simulink model "IIR"  (R2025a)
settings: Solver=ode45  StartTime=0.0  StopTime=10000  RelTol=1e-3  EnableMultiTasking=on
PreLoadFcn:
  | IIR_PreLoadFcn
undefined symbols (not defined in the file): num_channels, S, vsva2197, xcvc1902
libraries: hdlBasic x124, hdlUtilities x1, vmcUtilities x1
settings Model: Creator=alexc  LastModifiedBy=robg
settings SolverCC: AlgebraicLoopSolver=TrustRegion
settings DataIOCC: LimitDataPoints=on  SaveFormat=Array  SignalLoggingSaveFormat=ModelDataLogs  ReturnWorkspaceOutputs=off  SignalLoggingName=sigsOut
settings OptimizationCC: BlockReduction=off  BooleanDataType=off  DefaultParameterBehavior=Inlined  ExpressionDepthLimit=2147483647.0  InitFltsAndDblsToZero=on  LifeSpan=inf
settings DebuggingCC: SaveWithParameterizedLinksMsg=none  UnderspecifiedInitializationDetection=Classic  MergeDetectMultiDrivingBlocksExec=none  SignalResolutionControl=TryResolveAllWithWarning  MultiTaskDSMMsg=warning  MultiTaskCondExecSysMsg=none  FcnCallInpInsideContextMsg=warning  UnconnectedInputMsg=warning  UnconnectedOutputMsg=warning  UnconnectedLineMsg=warning  AllowSymbolicDim=off  StateNameClashWarn=warning  SFUnexpectedBacktrackingDiag=warning  SFNoUnconditionalDefaultTransitionDiag=warning  SFExecutionAtInitializationDiag=none  ArithmeticOperatorsInVariantConditions=warning
settings HardwareCC: ProdBitPerPointer=32.0  ProdBitPerSizeT=32.0  ProdBitPerPtrDiffT=32.0  ProdLargestAtomicFloat=None  ProdIntDivRoundTo=Undefined  ProdEndianess=Unspecified  ProdWordSize=32.0  ProdHWDeviceType=32-bit Generic  TargetUnknown=on
settings ModelReferenceCC: EnableRefExpFcnMdlSchedulingChecks=on  PropagateSignalLabelsOutOfModel=off
settings SFSimCC: SimUseLocalCustomCode=off  CustomCodeUndefinedFunction=UseInterfaceOnly
settings RTWCC: RTWUseLocalCustomCode=off  GPUComputeCapability=3.5  DLArmComputeVersion=19.05
settings CodeAppCC: StateflowObjectComments=on
settings GRTTargetCC: TargetFcnLib=ansi_tfl_tmw.mat  TargetLangStandard=C89/C90 (ANSI)  CombineOutputUpdateFcns=off  GRTInterface=on
settings ConfigComp: CovMetricSettings=dw  CovSaveCumulativeToWorkspaceVar=on  CovSaveSingleToWorkspaceVar=on  CovExternalEMLEnable=off

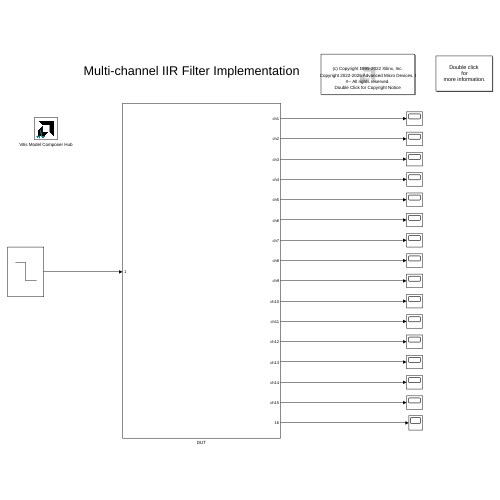
[thumbnail: Simulink's stored preview of the top-level diagram]
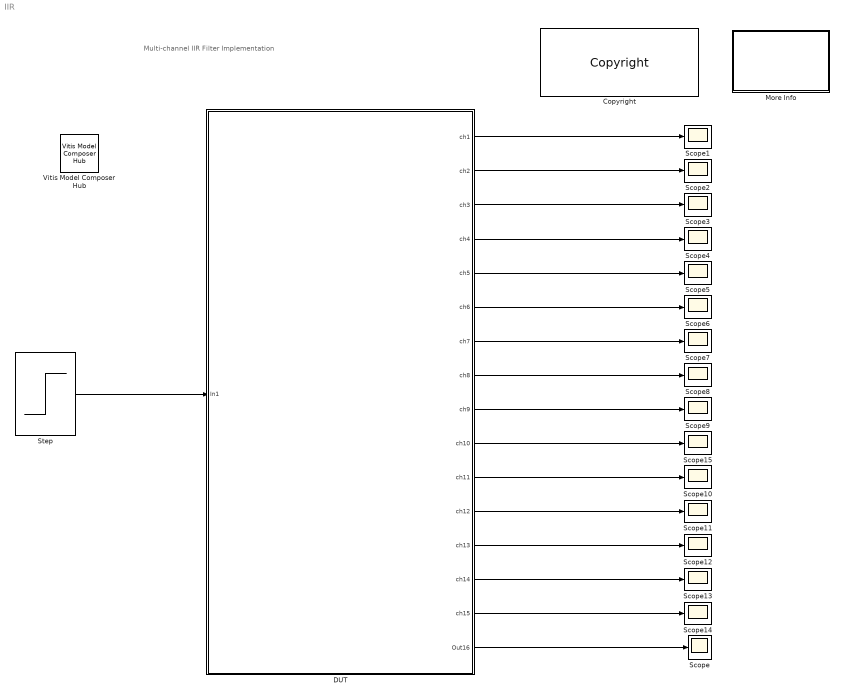
== system IIR ==
  note: Multi-channel IIR Filter Implementation
  Copyright : hdlUtilities/Copyright  copyrighttext="(c) Copyright 1995-2022 Xilinx, Inc. <br>(c) Copyright 2022-2026 Advanced Micro Devices, Inc. All rights reserved.<br><br>This document  contains proprietary, confidential information that may be used, copied and/or disclosed only as authorized by a valid licensing agreement with Advanced Micro Devices, Inc. This copyright notice must be retained on all authorized copies.<br><br> This code is provided \"as is\". Advanced Micro Devices, Inc. makes, and the end user receives, no warranties or conditions, express, implied, statutory or otherwise, and Advanced Micro Devices, Inc. specifically disclaims any implied warranties of merchantability, <br>non-infringement, or fitness for a particular purpose."  block_type=copyright
  DUT : Subsystem
  More Info : Subsystem
      mask Display: disp('Double click\n for\n more information.')
  Scope{,1..15} (16 alike) : Scope
      Scope settings: DataLoggingVariableName=ScopeData15
      Scope1 settings: ActiveDisplayYMinimum=-1  ActiveDisplayYMaximum=1
      Scope10 settings: DataLoggingVariableName=ScopeData2
      Scope11 settings: DataLoggingVariableName=ScopeData3
      Scope12 settings: DataLoggingVariableName=ScopeData4
      Scope13 settings: ActiveDisplayYMinimum=0.425  ActiveDisplayYMaximum=0.65  DataLoggingVariableName=ScopeData5
      Scope14 settings: ActiveDisplayYMinimum=0.39  ActiveDisplayYMaximum=0.51  DataLoggingVariableName=ScopeData6
      Scope15 settings: DataLoggingVariableName=ScopeData7
      Scope2 settings: DataLoggingVariableName=ScopeData8
      Scope3 settings: DataLoggingVariableName=ScopeData9
      Scope4 settings: DataLoggingVariableName=ScopeData10
      Scope5 settings: DataLoggingVariableName=ScopeData11
      Scope6 settings: DataLoggingVariableName=ScopeData12
      Scope7 settings: DataLoggingVariableName=ScopeData13
      Scope8 settings: DataLoggingVariableName=ScopeData14
  Step : Step  Time=300  Before=1  After=0  SampleTime=5
  Vitis Model Composer Hub : vmcUtilities/Vitis Model Composer Hub  Tag=genX  CodeGeneration=off  SubsystemName=DUT  BlockHierPath=IIR/DUT  CompilationType=HDLCompilation  SubsystemType=HDLNode  ExportTypeV2=IP Catalog  StartColumn=1  NumberOfColumns=1  TargetDirectory=./netlist  exportDesign=on  analyzeDesign=off  validateDesignOnHw=off  ExportType=System Generator  IpVendor=xilinx.com  IpLibrary=hls  IpVersion=1.0  IpHWLanguage=Verilog  AieCompilerOptions={}  AieSimulatorOptions={}  CreateTestbench=off  TestbenchStackSize=10  RunRtlSim=off  RunCSim=off  RunAieSim=off  enableSimulationTimeout=on  enableGraphIterations=on  AieSimTimeout=50000  AieGraphIterations=-1  RunAieSimProfiling=off  LaunchVitisAnalyzer=off  PlotOutput=off  RunX86Sim=off  X86SimTimeout=10  GenHwImage=off  GenLibadfXo=on  GenHwValidationCode=off  PlatformType=Not Specified  HwSystemType=Baremetal  HwValidationTarget=hw  ProjDevice=xcvc1902-vsva2197-1LP-e-S  ProjDevicePart=xcvc1902-vsva2197-1LP-e-S  AIEType=AIE  SamplePeriod=-1  ClockFrequency=200  DataPathParallelism=1  xilinxfamily=versalaicore  part=xcvc1902  speed=-1LP-e-S  package=vsva2197  directory=./netlist/ip/DUT/src  testbench=off  incr_netlist=off  synthesis_tool=Vivado  clock_wrapper=Clock Enables  dbl_ovrd=According to Block Masks  dcm_input_clock_period=10  sysclk_period=22  simulink_period=1  eval_field=0  IPInfoJsonString="{\"DUTSubsystemName\":\"DUT\",\"HDLSubsystem\":{\"SubsystemName\":\"DUT\",\"IPName\":\"Subsystem\",\"IPLibrary\":\"VMC\",\"IPVendor\":\"User Company\",\"IPVersion\":\"1.0\",\"TargetDirectory\":\"./netlist\",\"SubsystemDir\":\"./netlist/ip/DUT\",\"FreqHz\":\"45454545.4545\"},\"SubsystemTag\":\"HDLNode\"}"  LogFileName=/proj/xhdhdstaff5/sdegala/Head1/HEAD/ModelComposer_Sept16/Vitis_Model_Composer/Examples/HDL/Digital_Filtering/Multi_Channel_Folded_impl/netlist/model_composer.log  NThreads=4  IPConfigFile=/tmp/vmctmp-9769773316677438567/IIR_ipconfig.json
  wires:
  Step/1 -> DUT/1(In1)
  DUT/1(ch1) -> Scope1/1
  DUT/2(ch2) -> Scope2/1
  DUT/3(ch3) -> Scope3/1
  DUT/4(ch4) -> Scope4/1
  DUT/5(ch5) -> Scope5/1
  DUT/6(ch6) -> Scope6/1
  DUT/7(ch7) -> Scope7/1
  DUT/8(ch8) -> Scope8/1
  DUT/9(ch9) -> Scope9/1
  DUT/10(ch10) -> Scope15/1
  DUT/11(ch11) -> Scope10/1
  DUT/12(ch12) -> Scope11/1
  DUT/13(ch13) -> Scope12/1
  DUT/14(ch14) -> Scope13/1
  DUT/15(ch15) -> Scope14/1
  DUT/16(Out16) -> Scope/1

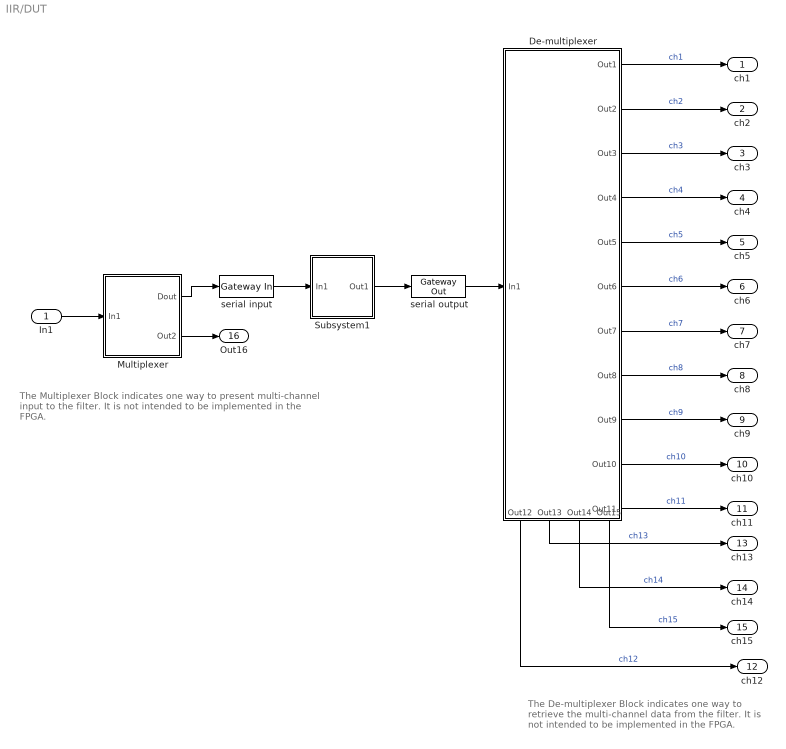
== system IIR/DUT ==
  note: The Multiplexer Block indicates one way to present
      | multi-channel input to the filter.  It is not intended to
      | be implemented in the FPGA.
  note: The De-multiplexer Block indicates one
      | way to retrieve the multi-channel data
      | from the filter. It is not intended to be
      | implemented in the FPGA.
  In1 : Inport
  De-multiplexer : Subsystem
      settings: PortSchema="{\"entries\":[{\"content\":{\"sides\":[{\"content\":{\"connectorIds\":[\"In1\"]},\"type\":\"ConnectorPlacement.EquallySpacedRectSide\",\"uuid\":\"3b4ff2fd-50a8-43bd-9bae-2460b1030825\"},{\"content\":{\"connectorIds\":[\"Out1\",\"Out2\",\"Out3\",\"Out4\",\"Out5\",\"Out6\",\"Out7\",\"Out8\",\"Out9\",\"Out10\",\"Out11\"],\"side\":\"RIGHT\"},\"type\":\"ConnectorPlacement.EquallySpacedRectSide\",\"uuid\":\"e1c9733d-22c8-4d91-9bdb-dd885a91145e\"},{\"content\":{\"connectorIds\":[],\"side\":\"TOP\"},\"type\":\"ConnectorPlacement.EquallySpacedRectSide\",\"uuid\":\"9c55e95b-c644-4887-b540-85aa80116050\"},{\"content\":{\"connectorIds\":[\"Out12\",\"Out13\",\"Out14\",\"Out15\"],\"side\":\"BOTTOM\"},\"type\":\"ConnectorPlacement.EquallySpacedRectSide\",\"uuid\":\"c33d5f17-02c8-4636-8e06-dc6f6aaa12a1\"}]},\"type\":\"ConnectorPlacement.EquallySpacedConnector\",\"uuid\":\"c0c50374-cd7b-45fa-b9e9-8e15c8f9419a\"}],\"packageUris\":[\"http://schema.mathworks.com/mf0/Connector/R2020b\"],\"version\":\"1.0\"}"
  Multiplexer : Subsystem
  Subsystem1 : Subsystem
  serial input : hdlBasic/Gateway In  gui_display_data_type=Fixed-point  arith_type=Signed (2's comp)  n_bits=data_width_nbits  bin_pt=data_width_frac  preci_type=Single  exp_width=8  frac_width=24  rows=1  columns=1  quantization="Round  (unbiased: +/- Inf)"  overflow=Saturate  period=5  UseAsADC=off  ADCChannel='1'  interface=None  automatic_assignment=on  address_offset=hex2dec('00')  intf_name=''  intf_description=''  default_value=0  timing_constraint=Data Rate  locs_specified=off  LOCs={}  io_standard={}  inherit_from_input=off  hdl_port=on  XmcBlockStatus=1  maskContainerNames=group4  block_type=gatewayin  block_config=sysgen:gateway_in_config  block_width_w=590  block_height_w=620  block_width=640  block_height=850
  serial output : hdlBasic/Gateway Out  inherit_from_input=off  bool_to_boolean=off  hdl_port=on  rows=1  columns=1  UseAsDAC=off  DACChannel='1'  interface=None  automatic_assignment=on  address_offset=hex2dec('00')  intf_name=''  intf_description=''  timing_constraint=Data Rate  locs_specified=off  LOCs={}  io_standard={}  XmcBlockStatus=1  maskContainerNames=group4  block_type=gatewayout  block_config=sysgen:gateway_out_config  block_width_w=590  block_height_w=620  block_width=620  block_height=750
  ch1 : Outport
  ch2 : Outport  Port=2
  ch3 : Outport  Port=3
  ch4 : Outport  Port=4
  ch5 : Outport  Port=5
  ch6 : Outport  Port=6
  ch7 : Outport  Port=7
  ch8 : Outport  Port=8
  ch9 : Outport  Port=9
  ch10 : Outport  Port=10
  ch11 : Outport  Port=11
  ch12 : Outport  Port=12
  ch13 : Outport  Port=13
  ch14 : Outport  Port=14
  ch15 : Outport  Port=15
  Out16 : Outport  Port=16
  wires:
  De-multiplexer/5(Out5) -> ch5/1  "ch5"
  De-multiplexer/15(Out15) -> ch15/1  "ch15"
  De-multiplexer/12(Out12) -> ch12/1  "ch12"
  De-multiplexer/6(Out6) -> ch6/1  "ch6"
  serial input/1 -> Subsystem1/1(In1)
  De-multiplexer/13(Out13) -> ch13/1  "ch13"
  De-multiplexer/7(Out7) -> ch7/1  "ch7"
  serial output/1 -> De-multiplexer/1(In1)
  De-multiplexer/4(Out4) -> ch4/1  "ch4"
  De-multiplexer/11(Out11) -> ch11/1  "ch11"
  Multiplexer/1(Dout) -> serial input/1
  De-multiplexer/10(Out10) -> ch10/1  "ch10"
  Subsystem1/1(Out1) -> serial output/1
  De-multiplexer/8(Out8) -> ch8/1  "ch8"
  De-multiplexer/14(Out14) -> ch14/1  "ch14"
  De-multiplexer/1(Out1) -> ch1/1  "ch1"
  In1/1 -> Multiplexer/1(In1)
  De-multiplexer/3(Out3) -> ch3/1  "ch3"
  De-multiplexer/9(Out9) -> ch9/1  "ch9"
  De-multiplexer/2(Out2) -> ch2/1  "ch2"
  Multiplexer/2(Out2) -> Out16/1

== system IIR/More Info ==
  note: This design demonstrates how multiple IIR filters can be implemented using a single time-shared second-order section (biquad).  Specifically,
      | 15 distinct IIR filters, each consisting of four cascaded biquads, are realized in a "folded" architecture that uses a single hardware biquad.
      | Hardware folding is a technique to time-multiplex many algorithm operations onto a single functional unit (e.g. adder, multiplier).   For low
      | sample rate applications like audio and control, the required silicon area can be much reduced by time-sharing the hardware resources.
      |
      | In this design, the several individual folding techniques are employed:
      |  - the biquad is time-multiplexed among fifteen channels
      |  - the biquad is time-multiplexed among four cascade stages for each channel
      |  - the biquad is implemented using two multipliers and a single adder instead of the straightforward 5 multipliers and 4 adders (a biquad output
      |    is calculated in every 5 system clock cycles).
  note: Multi-channel IIR Filter Implementation

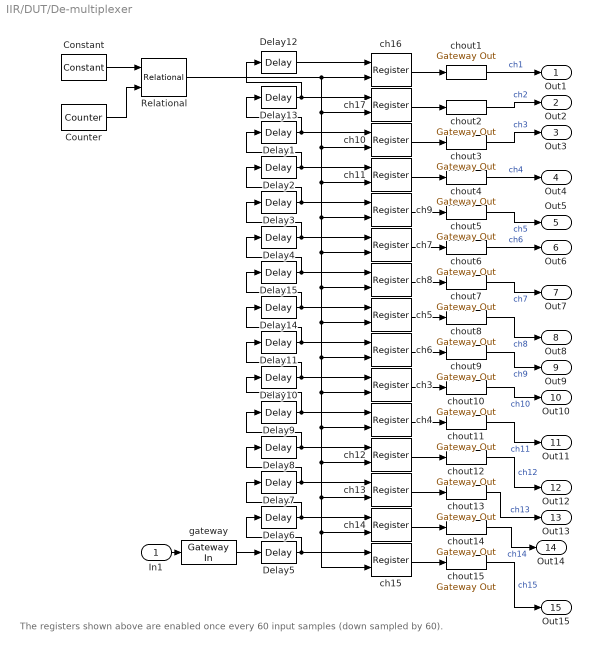
== system IIR/DUT/De-multiplexer ==
  note: The registers shown above are enabled once every 60 input samples (down sampled by 60).
  In1 : Inport
  Constant : hdlBasic/Constant  const=0  gui_display_data_type=Fixed-point  arith_type=Unsigned  n_bits=1  bin_pt=0  preci_type=Single  exp_width=8  frac_width=24  explicit_period=off  period=1  XmcBlockStatus=1  maskContainerNames=tabcontainer1  block_type=constant  block_config=sysgen:Constant_config
  Counter : hdlBasic/Counter  cnt_type=Count limited  cnt_to=4*num_channels-1  operation=Up  start_count=0  cnt_by_val=1  arith_type=Unsigned  n_bits=ceil(log2(4*num_channels))  bin_pt=0  load_pin=off  rst=off  en=off  explicit_period=Explicit  period=5  use_behavioral_HDL=off  implementation=Fabric  use_rpm=off  XmcBlockStatus=1  maskContainerNames=group1  block_type=counter  block_config=sysgen:Counter_config  block_width=531  block_height=1023
  Delay{1..15} (15 alike) : hdlBasic/Delay  rst=off  en=off  latency=1  reg_retiming=off  XmcBlockStatus=1  maskContainerNames=group1  block_type=delay  block_config=sysgen:Delay_config
  Relational : hdlBasic/Relational  mode=a=b  op_type=Bool  en=off  latency=0  XmcBlockStatus=1  maskContainerNames=tabcontainer1  block_type=relational  block_config=sysgen:Relational_config
  ch{3..17} (15 alike) : hdlBasic/Register  init=0  rst=off  en=on  XmcBlockStatus=1  maskContainerNames=tabcontainer1  block_type=register  block_config=sysgen:Register_config
  chout{1..15} (15 alike) : hdlBasic/Gateway Out  inherit_from_input=off  bool_to_boolean=off  hdl_port=off  rows=1  columns=1  UseAsDAC=off  DACChannel='1'  interface=None  automatic_assignment=on  address_offset=hex2dec('00')  intf_name=''  intf_description=''  timing_constraint=Data Rate  locs_specified=off  LOCs={}  io_standard={}  XmcBlockStatus=1  maskContainerNames=group4  block_type=gatewayout  block_config=sysgen:gateway_out_config  block_width_w=590  block_height_w=620  block_width=620  block_height=750
  gateway : hdlBasic/Gateway In  gui_display_data_type=Fixed-point  arith_type=Signed (2's comp)  n_bits=data_width_nbits  bin_pt=data_width_frac  preci_type=Single  exp_width=8  frac_width=24  rows=1  columns=1  quantization="Round  (unbiased: +/- Inf)"  overflow=Saturate  period=5  UseAsADC=off  ADCChannel='1'  interface=None  automatic_assignment=on  address_offset=hex2dec('00')  intf_name=''  intf_description=''  default_value=0  timing_constraint=Data Rate  locs_specified=off  LOCs={}  io_standard={}  inherit_from_input=off  hdl_port=on  XmcBlockStatus=1  maskContainerNames=group4  block_type=gatewayin  block_config=sysgen:gateway_in_config  block_width_w=590  block_height_w=620  block_width=640  block_height=850
  Out1 : Outport
  Out2 : Outport  Port=2
  Out3 : Outport  Port=3
  Out4 : Outport  Port=4
  Out5 : Outport  Port=5
  Out6 : Outport  Port=6
  Out7 : Outport  Port=7
  Out8 : Outport  Port=8
  Out9 : Outport  Port=9
  Out10 : Outport  Port=10
  Out11 : Outport  Port=11
  Out12 : Outport  Port=12
  Out13 : Outport  Port=13
  Out14 : Outport  Port=14
  Out15 : Outport  Port=15
  wires:
  Counter/1 -> Relational/2
  Constant/1 -> Relational/1
  gateway/1 -> Delay5/1
  Delay4/1 -> ch7/1, Delay3/1
  Delay3/1 -> ch9/1, Delay2/1
  Delay2/1 -> ch11/1, Delay1/1
  Delay1/1 -> ch10/1, Delay13/1
  Delay13/1 -> ch17/1, Delay12/1
  Delay12/1 -> ch16/1
  ch16/1 -> chout1/1
  ch17/1 -> chout2/1
  ch10/1 -> chout3/1
  ch11/1 -> chout4/1
  ch9/1 -> chout5/1
  ch7/1 -> chout6/1
  ch8/1 -> chout7/1
  ch5/1 -> chout8/1
  ch6/1 -> chout9/1
  ch3/1 -> chout10/1
  ch4/1 -> chout11/1
  ch12/1 -> chout12/1
  ch13/1 -> chout13/1
  ch14/1 -> chout14/1
  ch15/1 -> chout15/1
  In1/1 -> gateway/1
  Relational/1 -> ch15/2, ch14/2, ch13/2, ch12/2, ch4/2, ch3/2, ch6/2, ch5/2, ch8/2, ch7/2, ch9/2, ch11/2, ch10/2, ch17/2, ch16/2
  Delay5/1 -> Delay6/1, ch15/1
  Delay6/1 -> ch14/1, Delay7/1
  Delay7/1 -> ch13/1, Delay8/1
  Delay8/1 -> ch12/1, Delay9/1
  Delay9/1 -> ch4/1, Delay10/1
  Delay10/1 -> ch3/1, Delay11/1
  Delay11/1 -> ch6/1, Delay14/1
  Delay14/1 -> ch5/1, Delay15/1
  Delay15/1 -> ch8/1, Delay4/1
  chout1/1 -> Out1/1  "ch1"
  chout2/1 -> Out2/1  "ch2"
  chout3/1 -> Out3/1  "ch3"
  chout4/1 -> Out4/1  "ch4"
  chout5/1 -> Out5/1  "ch5"
  chout7/1 -> Out7/1  "ch7"
  chout6/1 -> Out6/1  "ch6"
  chout8/1 -> Out8/1  "ch8"
  chout9/1 -> Out9/1  "ch9"
  chout10/1 -> Out10/1  "ch10"
  chout11/1 -> Out11/1  "ch11"
  chout12/1 -> Out12/1  "ch12"
  chout13/1 -> Out13/1  "ch13"
  chout14/1 -> Out14/1  "ch14"
  chout15/1 -> Out15/1  "ch15"

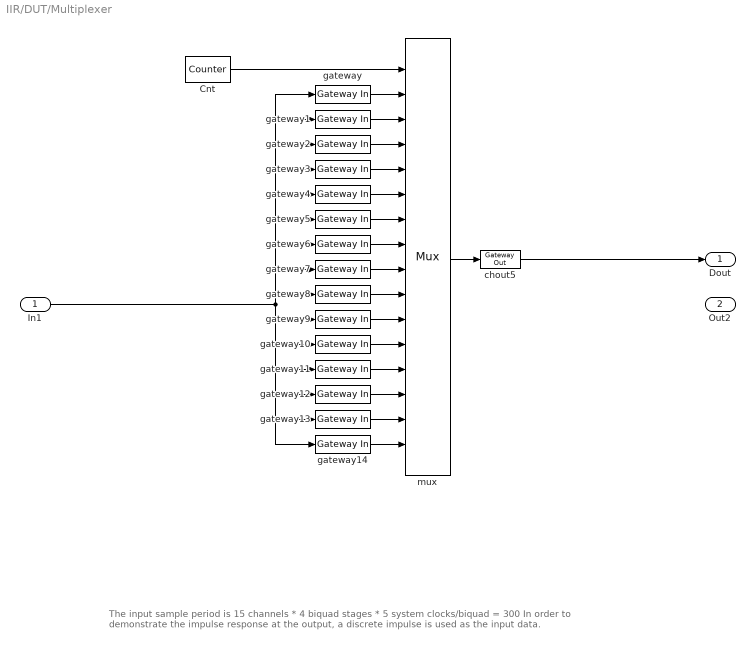
== system IIR/DUT/Multiplexer ==
  note: The input sample period is 15 channels * 4 biquad stages * 5 system clocks/biquad = 300
      | In order to demonstrate the impulse response at the output, a discrete impulse is used as
      | the input data.
  In1 : Inport
  Cnt : hdlBasic/Counter  cnt_type=Count limited  cnt_to=num_channels-1  operation=Up  start_count=0  cnt_by_val=1  arith_type=Unsigned  n_bits=ceil(log2(num_channels))  bin_pt=0  load_pin=off  rst=off  en=off  explicit_period=Explicit  period=5  use_behavioral_HDL=off  implementation=Fabric  use_rpm=off  XmcBlockStatus=1  maskContainerNames=group1  block_type=counter  block_config=sysgen:Counter_config  block_width=531  block_height=1023
  chout5 : hdlBasic/Gateway Out  inherit_from_input=off  bool_to_boolean=off  hdl_port=off  rows=1  columns=1  UseAsDAC=off  DACChannel='1'  interface=None  automatic_assignment=on  address_offset=hex2dec('00')  intf_name=''  intf_description=''  timing_constraint=Data Rate  locs_specified=off  LOCs={}  io_standard={}  XmcBlockStatus=1  maskContainerNames=group4  block_type=gatewayout  block_config=sysgen:gateway_out_config  block_width_w=590  block_height_w=620  block_width=620  block_height=750
  gateway{,1..14} (15 alike) : hdlBasic/Gateway In  gui_display_data_type=Fixed-point  arith_type=Signed (2's comp)  n_bits=data_width_nbits  bin_pt=data_width_frac  preci_type=Single  exp_width=8  frac_width=24  rows=1  columns=1  quantization="Round  (unbiased: +/- Inf)"  overflow=Saturate  period=5  UseAsADC=off  ADCChannel='1'  interface=None  automatic_assignment=on  address_offset=hex2dec('00')  intf_name=''  intf_description=''  default_value=0  timing_constraint=Data Rate  locs_specified=off  LOCs={}  io_standard={}  inherit_from_input=off  hdl_port=on  XmcBlockStatus=1  maskContainerNames=group4  block_type=gatewayin  block_config=sysgen:gateway_in_config  block_width_w=590  block_height_w=620  block_width=640  block_height=850
  mux : hdlBasic/Mux  inputs=15  en=off  latency=0  precision=Full  arith_type="Signed  (2's comp)"  n_bits=8  bin_pt=2  quantization=Truncate  overflow=Wrap  XmcBlockStatus=1  maskContainerNames=tabcontainer1  block_type=mux  block_config=sysgen:Mux_config
  Dout : Outport  VectorParamsAs1DForOutWhenUnconnected=off
  Out2 : Outport  Port=2
  wires:
  mux/1 -> chout5/1
  chout5/1 -> Dout/1
  gateway/1 -> mux/2
  gateway1/1 -> mux/3
  gateway2/1 -> mux/4
  gateway3/1 -> mux/5
  gateway4/1 -> mux/6
  gateway5/1 -> mux/7
  gateway6/1 -> mux/8
  gateway7/1 -> mux/9
  gateway8/1 -> mux/10
  gateway9/1 -> mux/11
  gateway10/1 -> mux/12
  gateway11/1 -> mux/13
  gateway12/1 -> mux/14
  gateway13/1 -> mux/15
  gateway14/1 -> mux/16
  In1/1 -> gateway/1, gateway1/1, gateway2/1, gateway3/1, gateway4/1, gateway5/1, gateway6/1, gateway7/1, gateway8/1, gateway9/1, gateway10/1, gateway11/1, gateway12/1, gateway13/1, gateway14/1
  Cnt/1 -> mux/1

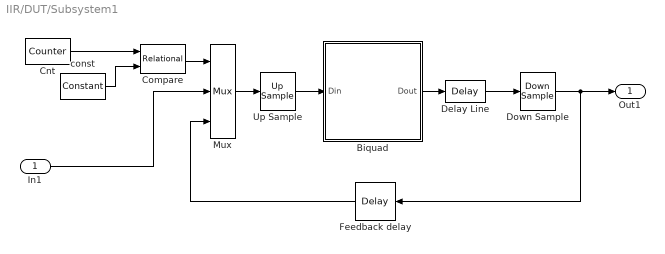
== system IIR/DUT/Subsystem1 ==
  In1 : Inport
  Biquad : Subsystem
  Cnt : hdlBasic/Counter  cnt_type=Count limited  cnt_to=4*num_channels-1  operation=Up  start_count=0  cnt_by_val=1  arith_type=Unsigned  n_bits=ceil(log2(4*num_channels))  bin_pt=0  load_pin=off  rst=off  en=off  explicit_period=Explicit  period=5  use_behavioral_HDL=off  implementation=Fabric  use_rpm=off  XmcBlockStatus=1  maskContainerNames=group1  block_type=counter  block_config=sysgen:Counter_config  block_width=531  block_height=1023
  Compare : hdlBasic/Relational  mode=a>b  op_type=Bool  en=off  latency=0  XmcBlockStatus=1  maskContainerNames=tabcontainer1  block_type=relational  block_config=sysgen:Relational_config
  Delay Line : hdlBasic/Delay  rst=off  en=off  latency=3  reg_retiming=off  XmcBlockStatus=1  maskContainerNames=group1  block_type=delay  block_config=sysgen:Delay_config
  Down Sample : hdlBasic/Down Sample  sample_ratio=5  sample_phase=First Value of Frame  en=off  rst=off  latency=0  XmcBlockStatus=1  maskContainerNames=group1  block_type=dsamp  block_config=sysgen:Downsample_config
  Feedback delay : hdlBasic/Delay  rst=off  en=off  latency=14  reg_retiming=off  XmcBlockStatus=1  maskContainerNames=group1  block_type=delay  block_config=sysgen:Delay_config
  Mux : hdlBasic/Mux  inputs=2  en=off  latency=0  precision=Full  arith_type="Signed  (2's comp)"  n_bits=8  bin_pt=2  quantization=Truncate  overflow=Wrap  XmcBlockStatus=1  maskContainerNames=tabcontainer1  block_type=mux  block_config=sysgen:Mux_config
  Up Sample : hdlBasic/Up Sample  sample_ratio=5  copy_samples=off  en=off  latency=0  XmcBlockStatus=1  maskContainerNames=group1  block_type=usamp  block_config=sysgen:Upsample_config
  const : hdlBasic/Constant  const=num_channels-1  gui_display_data_type=Fixed-point  arith_type=Unsigned  n_bits=ceil(log2(4*num_channels))  bin_pt=0  preci_type=Single  exp_width=8  frac_width=24  explicit_period=off  period=1  XmcBlockStatus=1  maskContainerNames=tabcontainer1  block_type=constant  block_config=sysgen:Constant_config
  Out1 : Outport
  wires:
  Biquad/1(Dout) -> Delay Line/1
  In1/1 -> Mux/2
  Delay Line/1 -> Down Sample/1
  Up Sample/1 -> Biquad/1(Din)
  Down Sample/1 -> Out1/1, Feedback delay/1
  Mux/1 -> Up Sample/1
  Feedback delay/1 -> Mux/3
  Compare/1 -> Mux/1
  Cnt/1 -> Compare/1
  const/1 -> Compare/2

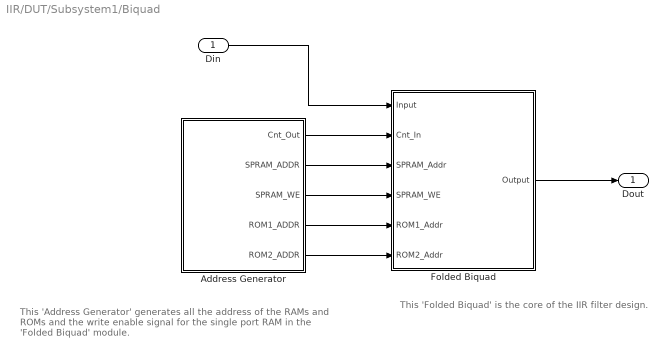
== system IIR/DUT/Subsystem1/Biquad ==
  note: This 'Address Generator' generates all the address of the
      | RAMs and ROMs and the write enable signal for the single
      | port RAM in the 'Folded Biquad' module.
  note: This 'Folded Biquad' is the core of the IIR filter design.
  Din : Inport
  Address Generator : Subsystem
  Folded Biquad : Subsystem
  Dout : Outport  VectorParamsAs1DForOutWhenUnconnected=off
  wires:
  Address Generator/1(Cnt_Out) -> Folded Biquad/2(Cnt_In)
  Address Generator/2(SPRAM_ADDR) -> Folded Biquad/3(SPRAM_Addr)
  Address Generator/3(SPRAM_WE) -> Folded Biquad/4(SPRAM_WE)
  Address Generator/4(ROM1_ADDR) -> Folded Biquad/5(ROM1_Addr)
  Address Generator/5(ROM2_ADDR) -> Folded Biquad/6(ROM2_Addr)
  Folded Biquad/1(Output) -> Dout/1
  Din/1 -> Folded Biquad/1(Input)

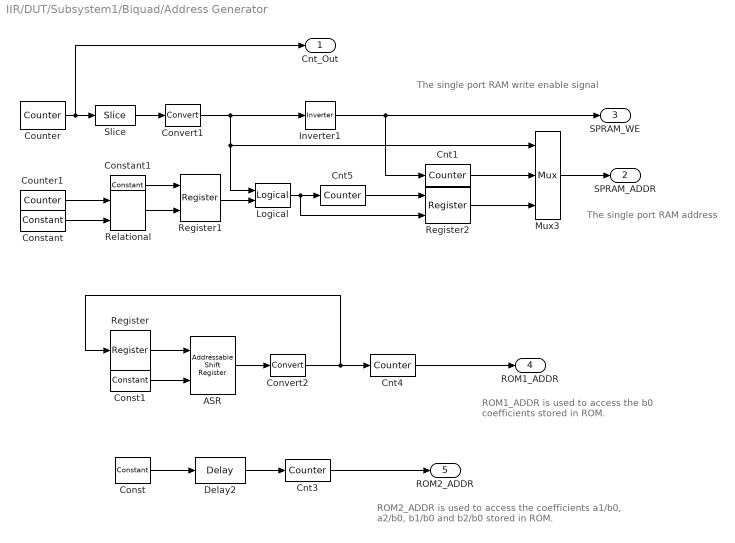
== system IIR/DUT/Subsystem1/Biquad/Address Generator ==
  note: ROM1_ADDR is used to access
      | the b0 coefficients stored in ROM.
  note: ROM2_ADDR is used to access  the coefficients
      | a1/b0, a2/b0, b1/b0 and b2/b0 stored in ROM.
  note: The single port RAM address
  note: The single port RAM write enable signal
  ASR : hdlBasic/Addressable Shift Register  infer_latency=on  depth=4  initVector=[0 0 0 0]  en=off  use_behavioral_HDL=off  Optimization=Resource  use_rpm=off  XmcBlockStatus=1  maskContainerNames=group1  block_type=addrsr  block_config=sysgen:Addrsr_config
  Cnt1 : hdlBasic/Counter  cnt_type=Count limited  cnt_to=16*num_channels-1  operation=Up  start_count=0  cnt_by_val=1  arith_type=Unsigned  n_bits=bits_needed_3  bin_pt=0  load_pin=off  rst=off  en=on  explicit_period=Inferred from inputs  period=1  use_behavioral_HDL=off  implementation=Fabric  use_rpm=off  XmcBlockStatus=1  maskContainerNames=group1  block_type=counter  block_config=sysgen:Counter_config  block_width=531  block_height=1023
  Cnt3 : hdlBasic/Counter  cnt_type=Count limited  cnt_to=20*num_channels-1  operation=Up  start_count=0  cnt_by_val=1  arith_type=Unsigned  n_bits=bits_needed_2  bin_pt=0  load_pin=off  rst=off  en=on  explicit_period=Explicit  period=1  use_behavioral_HDL=off  implementation=Fabric  use_rpm=off  XmcBlockStatus=1  maskContainerNames=group1  block_type=counter  block_config=sysgen:Counter_config  block_width=531  block_height=1023
  Cnt4 : hdlBasic/Counter  cnt_type=Count limited  cnt_to=4*num_channels-1  operation=Up  start_count=0  cnt_by_val=1  arith_type=Unsigned  n_bits=bits_needed_1  bin_pt=0  load_pin=off  rst=off  en=on  explicit_period=Explicit  period=1  use_behavioral_HDL=off  implementation=Fabric  use_rpm=off  XmcBlockStatus=1  maskContainerNames=group1  block_type=counter  block_config=sysgen:Counter_config  block_width=531  block_height=1023
  Cnt5 : hdlBasic/Counter  cnt_type=Count limited  cnt_to=16*num_channels-1  operation=Up  start_count=3  cnt_by_val=4  arith_type=Unsigned  n_bits=bits_needed_3  bin_pt=0  load_pin=off  rst=off  en=on  explicit_period=Inferred from inputs  period=1  use_behavioral_HDL=off  implementation=Fabric  use_rpm=off  XmcBlockStatus=1  maskContainerNames=group1  block_type=counter  block_config=sysgen:Counter_config  block_width=531  block_height=1023
  Const : hdlBasic/Constant  const=1  gui_display_data_type=Boolean  arith_type=Boolean  n_bits=1  bin_pt=0  preci_type=Single  exp_width=8  frac_width=24  explicit_period=on  period=1  XmcBlockStatus=1  maskContainerNames=tabcontainer1  block_type=constant  block_config=sysgen:Constant_config
  Const1 : hdlBasic/Constant  const=3  gui_display_data_type=Fixed-point  arith_type=Unsigned  n_bits=2  bin_pt=0  preci_type=Single  exp_width=8  frac_width=24  explicit_period=on  period=1  XmcBlockStatus=1  maskContainerNames=tabcontainer1  block_type=constant  block_config=sysgen:Constant_config
  Constant : hdlBasic/Constant  const=20*num_channels-7  gui_display_data_type=Fixed-point  arith_type=Unsigned  n_bits=9  bin_pt=0  preci_type=Single  exp_width=8  frac_width=24  explicit_period=off  period=1  XmcBlockStatus=1  maskContainerNames=tabcontainer1  block_type=constant  block_config=sysgen:Constant_config
  Constant1 : hdlBasic/Constant  const=1  gui_display_data_type=Boolean  arith_type=Boolean  n_bits=9  bin_pt=0  preci_type=Single  exp_width=8  frac_width=24  explicit_period=off  period=1  XmcBlockStatus=1  maskContainerNames=tabcontainer1  block_type=constant  block_config=sysgen:Constant_config
  Convert1 : hdlBasic/Convert  gui_display_data_type=Boolean  arith_type=Boolean  n_bits=8  bin_pt=6  float_type=Single  exp_bits=8  fraction_bits=24  quantization=Truncate  overflow=Wrap  en=off  latency=0  pipeline=off  XmcBlockStatus=1  maskContainerNames=group2  block_type=convert  block_config=sysgen:Convert_config  block_width=595  block_height=885
  Convert2 : hdlBasic/Convert  gui_display_data_type=Boolean  arith_type=Boolean  n_bits=8  bin_pt=6  float_type=Single  exp_bits=8  fraction_bits=24  quantization=Truncate  overflow=Wrap  en=off  latency=0  pipeline=off  XmcBlockStatus=1  maskContainerNames=group2  block_type=convert  block_config=sysgen:Convert_config  block_width=595  block_height=885
  Counter : hdlBasic/Counter  cnt_type=Count limited  cnt_to=4  operation=Up  start_count=0  cnt_by_val=1  arith_type=Unsigned  n_bits=3  bin_pt=0  load_pin=off  rst=off  en=off  explicit_period=Explicit  period=1  use_behavioral_HDL=off  implementation=Fabric  use_rpm=off  XmcBlockStatus=1  maskContainerNames=group1  block_type=counter  block_config=sysgen:Counter_config  block_width=531  block_height=1023
  Counter1 : hdlBasic/Counter  cnt_type=Free running  cnt_to=4  operation=Up  start_count=0  cnt_by_val=1  arith_type=Unsigned  n_bits=9  bin_pt=0  load_pin=off  rst=off  en=off  explicit_period=Explicit  period=1  use_behavioral_HDL=off  implementation=Fabric  use_rpm=off  XmcBlockStatus=1  maskContainerNames=group1  block_type=counter  block_config=sysgen:Counter_config  block_width=531  block_height=1023
  Delay2 : hdlBasic/Delay  rst=off  en=off  latency=20*num_channels-1  reg_retiming=off  XmcBlockStatus=1  maskContainerNames=group1  block_type=delay  block_config=sysgen:Delay_config
  Inverter1 : hdlBasic/Inverter  en=off  latency=0  XmcBlockStatus=1  maskContainerNames=group2  block_type=inv  block_config=sysgen:Inverter_config
  Logical : hdlBasic/Logical  logical_function=AND  inputs=2  en=off  latency=0  precision=Full  arith_type=Unsigned  n_bits=8  bin_pt=2  align_bp=on  overflow=[]  quantization=[]  XmcBlockStatus=1  maskContainerNames=tabcontainer1  block_type=logical  block_config=sysgen:Logical_config
  Mux3 : hdlBasic/Mux  inputs=2  en=off  latency=0  precision=User Defined  arith_type=Unsigned  n_bits=bits_needed_3  bin_pt=0  quantization=Truncate  overflow=Flag as error  XmcBlockStatus=1  maskContainerNames=tabcontainer1  block_type=mux  block_config=sysgen:Mux_config
  Register : hdlBasic/Register  init=1  rst=off  en=off  XmcBlockStatus=1  maskContainerNames=tabcontainer1  block_type=register  block_config=sysgen:Register_config
  Register1 : hdlBasic/Register  init=0  rst=off  en=on  XmcBlockStatus=1  maskContainerNames=tabcontainer1  block_type=register  block_config=sysgen:Register_config
  Register2 : hdlBasic/Register  init=0  rst=off  en=on  XmcBlockStatus=1  maskContainerNames=tabcontainer1  block_type=register  block_config=sysgen:Register_config
  Relational : hdlBasic/Relational  mode=a=b  op_type=Bool  en=off  latency=0  XmcBlockStatus=1  maskContainerNames=tabcontainer1  block_type=relational  block_config=sysgen:Relational_config
  Slice : hdlBasic/Slice  nbits=1  boolean_output=off  mode=Upper Bit Location + Width  bit1=0  base1=MSB of Input  bit0=0  base0=LSB of Input  XmcBlockStatus=1  maskContainerNames=group1  block_type=slice  block_config=sysgen:Slice_config
  Cnt_Out : Outport  VectorParamsAs1DForOutWhenUnconnected=off
  SPRAM_ADDR : Outport  Port=2  VectorParamsAs1DForOutWhenUnconnected=off
  SPRAM_WE : Outport  Port=3  VectorParamsAs1DForOutWhenUnconnected=off
  ROM1_ADDR : Outport  Port=4  VectorParamsAs1DForOutWhenUnconnected=off
  ROM2_ADDR : Outport  Port=5  VectorParamsAs1DForOutWhenUnconnected=off
  wires:
  Delay2/1 -> Cnt3/1
  Cnt3/1 -> ROM2_ADDR/1
  Const/1 -> Delay2/1
  Convert2/1 -> Register/1, Cnt4/1
  ASR/1 -> Convert2/1
  Register/1 -> ASR/1
  Const1/1 -> ASR/2
  Cnt4/1 -> ROM1_ADDR/1
  Inverter1/1 -> SPRAM_WE/1, Cnt1/1
  Convert1/1 -> Mux3/1, Logical/1, Inverter1/1
  Slice/1 -> Convert1/1
  Counter/1 -> Cnt_Out/1, Slice/1
  Mux3/1 -> SPRAM_ADDR/1
  Cnt1/1 -> Mux3/2
  Counter1/1 -> Relational/1
  Constant/1 -> Relational/2
  Relational/1 -> Register1/2
  Constant1/1 -> Register1/1
  Register1/1 -> Logical/2
  Logical/1 -> Cnt5/1, Register2/2
  Cnt5/1 -> Register2/1
  Register2/1 -> Mux3/3

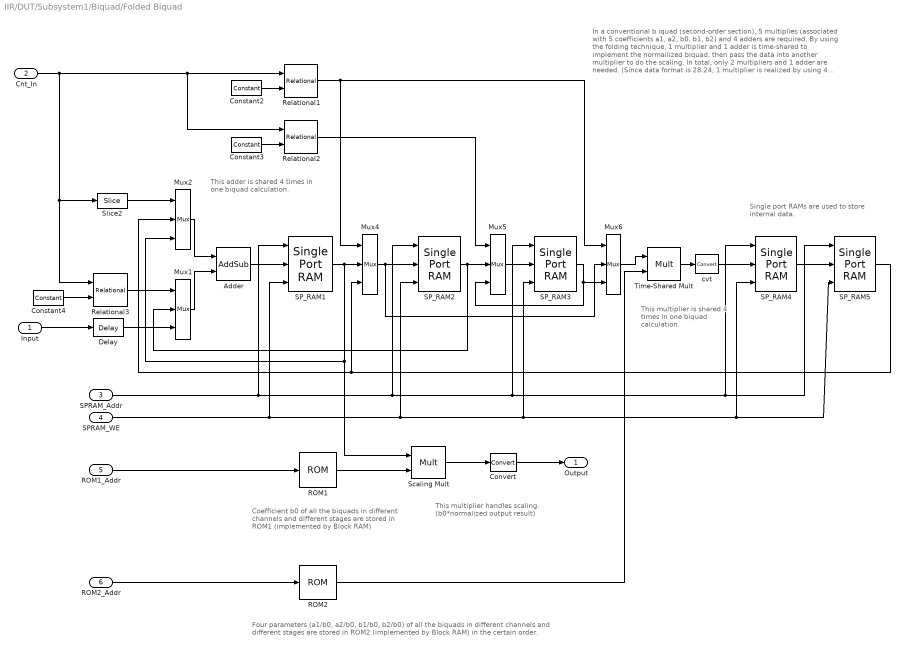
== system IIR/DUT/Subsystem1/Biquad/Folded Biquad ==
  note: Coefficient b0 of all the biquads in
      | different channels and different stages
      | are stored in ROM1 (implemented by
      | Block RAM)
  note: Four parameters (a1/b0, a2/b0, b1/b0, b2/b0) of all the biquads in different
      | channels and different stages are stored in ROM2 (implemented by Block RAM)
      | in the certain order.
  note: In a conventional b   iquad (second-order section), 5 multiplies
      | (associated with 5 coefficients a1, a2, b0, b1, b2) and 4 adders
      | are required.  By using the folding technique, 1 multiplier and
      | 1 adder is time-shared to implement the normailized biquad,
      | then pass the data into another multiplier to do the scaling.
      | In total, only 2 multipliers and 1 adder are needed. (Since
      | data format is 28.24, 1 multiplier is realized by using
      | 4 18x18 embedded multipliers )
  note: This multiplier is
      | shared 4 times in
      | one biquad
      | calculation.
  note: This adder is
      | shared 4 times
      | in one biquad
      | calculation.
  note: Single port RAMs are used to store
      | internal data.
  note: This multiplier handles scaling.
      | (b0*normalized output result)
  Input : Inport
  Cnt_In : Inport  Port=2
  SPRAM_Addr : Inport  Port=3
  SPRAM_WE : Inport  Port=4
  ROM1_Addr : Inport  Port=5
  ROM2_Addr : Inport  Port=6
  Adder : hdlBasic/AddSub  mode=Addition  use_carryin=off  use_carryout=off  en=off  latency=0  precision=User Defined  arith_type="Signed  (2's comp)"  n_bits=data_width_nbits  bin_pt=data_width_frac  quantization="Round  (unbiased: +/- Inf)"  overflow=Flag as error  use_behavioral_HDL=on  hw_selection=Fabric  pipelined=off  use_rpm=off  XmcBlockStatus=1  maskContainerNames=tabcontainer1  block_type=addsub  block_config=sysgen:Addsub_config
  Constant2 : hdlBasic/Constant  const=0  gui_display_data_type=Fixed-point  arith_type=Unsigned  n_bits=1  bin_pt=0  preci_type=Single  exp_width=8  frac_width=24  explicit_period=off  period=1  XmcBlockStatus=1  maskContainerNames=tabcontainer1  block_type=constant  block_config=sysgen:Constant_config
  Constant3 : hdlBasic/Constant  const=1  gui_display_data_type=Fixed-point  arith_type=Unsigned  n_bits=1  bin_pt=0  preci_type=Single  exp_width=8  frac_width=24  explicit_period=off  period=1  XmcBlockStatus=1  maskContainerNames=tabcontainer1  block_type=constant  block_config=sysgen:Constant_config
  Constant4 : hdlBasic/Constant  const=3  gui_display_data_type=Fixed-point  arith_type=Unsigned  n_bits=2  bin_pt=0  preci_type=Single  exp_width=8  frac_width=24  explicit_period=off  period=1  XmcBlockStatus=1  maskContainerNames=tabcontainer1  block_type=constant  block_config=sysgen:Constant_config
  Convert : hdlBasic/Convert  gui_display_data_type=Fixed-point  arith_type=Signed (2's comp)  n_bits=data_width_nbits  bin_pt=data_width_frac  float_type=Single  exp_bits=8  fraction_bits=24  quantization=Truncate  overflow=Wrap  en=off  latency=0  pipeline=off  XmcBlockStatus=1  maskContainerNames=group2  block_type=convert  block_config=sysgen:Convert_config  block_width=595  block_height=885
  Delay : hdlBasic/Delay  rst=off  en=off  latency=3  reg_retiming=off  XmcBlockStatus=1  maskContainerNames=group1  block_type=delay  block_config=sysgen:Delay_config
  Mux{1..2,4..6} (5 alike) : hdlBasic/Mux  inputs=2  en=off  latency=0  precision=User Defined  arith_type="Signed  (2's comp)"  n_bits=data_width_nbits  bin_pt=data_width_frac  quantization=Truncate  overflow=Flag as error  XmcBlockStatus=1  maskContainerNames=tabcontainer1  block_type=mux  block_config=sysgen:Mux_config
  ROM1 : hdlBasic/ROM  depth=4*num_channels  initVector=coeff_b0  distributed_mem=Block RAM  rst=off  init_reg=0  en=off  latency=2  gui_display_data_type=Fixed-point  arith_type="Signed  (2's comp)"  n_bits=data_width_nbits  bin_pt=data_width_frac  preci_type=Single  exp_width=8  frac_width=24  optimize=Area  use_rpm=off  simulation_type=fast_sim  XmcBlockStatus=1  maskContainerNames=tabcontainer1  block_type=sprom  block_config=sysgen:SPROM_config
  ROM2 : hdlBasic/ROM  depth=20*num_channels  initVector=coeffs  distributed_mem=Block RAM  rst=off  init_reg=0  en=off  latency=1  gui_display_data_type=Fixed-point  arith_type="Signed  (2's comp)"  n_bits=data_width_nbits  bin_pt=data_width_frac  preci_type=Single  exp_width=8  frac_width=24  optimize=Area  use_rpm=off  simulation_type=fast_sim  XmcBlockStatus=1  maskContainerNames=tabcontainer1  block_type=sprom  block_config=sysgen:SPROM_config
  Relational1 : hdlBasic/Relational  mode=a!=b  op_type=Bool  en=off  latency=0  XmcBlockStatus=1  maskContainerNames=tabcontainer1  block_type=relational  block_config=sysgen:Relational_config
  Relational2 : hdlBasic/Relational  mode=a!=b  op_type=Bool  en=off  latency=0  XmcBlockStatus=1  maskContainerNames=tabcontainer1  block_type=relational  block_config=sysgen:Relational_config
  Relational3 : hdlBasic/Relational  mode=a=b  op_type=Bool  en=off  latency=0  XmcBlockStatus=1  maskContainerNames=tabcontainer1  block_type=relational  block_config=sysgen:Relational_config
  SP_RAM{1..5} (5 alike) : hdlBasic/Single Port RAM  depth=16*num_channels  initVector=[zeros([1,16*num_channels])]  distributed_mem=Block RAM  write_mode=Read After Write  rst=off  init_reg=0  en=off  optimize_latency=off  latency=1  optimize=Area  dbl_ovrd=off  simulation_type=fast_sim  XmcBlockStatus=1  maskContainerNames=tabcontainer1  block_type=spram  block_config=sysgen:SPRAM_config
      SP_RAM2 settings: xl_area=[0 0 1 0 0 0 0]
      SP_RAM3 settings: xl_area=[0 0 1 0 0 0 0]
      SP_RAM4 settings: xl_area=[0 0 1 0 0 0 0]
      SP_RAM5 settings: xl_area=[0 0 1 0 0 0 0]
  Scaling Mult : hdlBasic/Mult  precision=User Defined  arith_type="Signed  (2's comp)"  n_bits=mult_width_nbits  bin_pt=mult_width_frac  quantization=Truncate  overflow=Flag as error  en=off  latency=0  opt_float=off  fp_mult_usage=No Usage  use_behavioral_HDL=off  opt=Speed  use_embedded=on  optimum_pipeline=off  pipeline=off  use_rpm=off  placement_style=Rectangular shape  XmcBlockStatus=1  maskContainerNames=group1  block_type=mult  block_config=sysgen:Mult_config  block_width=598  block_height=876
  Slice2 : hdlBasic/Slice  nbits=1  boolean_output=off  mode=Lower Bit Location + Width  bit1=0  base1=MSB of Input  bit0=0  base0=LSB of Input  XmcBlockStatus=1  maskContainerNames=group1  block_type=slice  block_config=sysgen:Slice_config
  Time-Shared Mult : hdlBasic/Mult  precision=Full  arith_type="Signed  (2's comp)"  n_bits=mult_width_nbits  bin_pt=mult_width_frac  quantization=Truncate  overflow=Flag as error  en=off  latency=0  opt_float=off  fp_mult_usage=No Usage  use_behavioral_HDL=off  opt=Speed  use_embedded=on  optimum_pipeline=off  pipeline=off  use_rpm=off  placement_style=Rectangular shape  XmcBlockStatus=1  maskContainerNames=group1  block_type=mult  block_config=sysgen:Mult_config  block_width=598  block_height=876
  cvt : hdlBasic/Convert  gui_display_data_type=Fixed-point  arith_type=Signed (2's comp)  n_bits=data_width_nbits  bin_pt=data_width_frac  float_type=Single  exp_bits=8  fraction_bits=24  quantization=Truncate  overflow=Wrap  en=off  latency=0  pipeline=off  XmcBlockStatus=1  maskContainerNames=group2  block_type=convert  block_config=sysgen:Convert_config  block_width=595  block_height=885
  Output : Outport  VectorParamsAs1DForOutWhenUnconnected=off
  wires:
  Time-Shared Mult/1 -> cvt/1
  Adder/1 -> SP_RAM1/2
  SP_RAM2/1 -> Mux5/2, Mux1/2
  Input/1 -> Delay/1
  Mux4/1 -> Mux6/2, SP_RAM2/2
  Mux5/1 -> SP_RAM3/2
  SP_RAM3/1 -> Mux6/3, Mux5/3
  cvt/1 -> SP_RAM4/2
  Delay/1 -> Mux1/3
  SP_RAM4/1 -> SP_RAM5/2
  Cnt_In/1 -> Relational1/1, Relational2/1, Relational3/1, Slice2/1
  SP_RAM1/1 -> Mux4/2, Mux2/3, Scaling Mult/1
  Constant2/1 -> Relational1/2
  Constant3/1 -> Relational2/2
  Relational2/1 -> Mux5/1
  Mux2/1 -> Adder/1
  Mux1/1 -> Adder/2
  Constant4/1 -> Relational3/2
  Relational3/1 -> Mux1/1
  Mux6/1 -> Time-Shared Mult/1
  SP_RAM5/1 -> Mux2/2, Mux4/3
  Slice2/1 -> Mux2/1
  ROM2/1 -> Time-Shared Mult/2
  Relational1/1 -> Mux4/1, Mux6/1
  Scaling Mult/1 -> Convert/1
  Convert/1 -> Output/1
  ROM1/1 -> Scaling Mult/2
  SPRAM_Addr/1 -> SP_RAM5/1, SP_RAM4/1, SP_RAM3/1, SP_RAM2/1, SP_RAM1/1
  SPRAM_WE/1 -> SP_RAM2/3, SP_RAM5/3, SP_RAM4/3, SP_RAM3/3, SP_RAM1/3
  ROM2_Addr/1 -> ROM2/1
  ROM1_Addr/1 -> ROM1/1
